simulink model "Cau3"  (R2021b)
settings: Solver=VariableStepAuto  StartTime=0.0  StopTime=inf  RelTol=1e-3
libraries: commsink2 x2, commutil2 x2, commdigbbndpm3 x2, commchan3 x1, commrandsrc3 x1
settings Model: Creator=ICTLAB  LastModifiedBy=ICTLAB
settings DataIOCC: ReturnWorkspaceOutputs=off

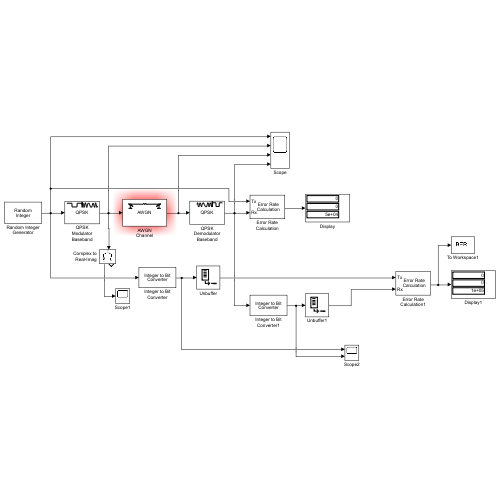
[thumbnail: Simulink's stored preview of the top-level diagram]
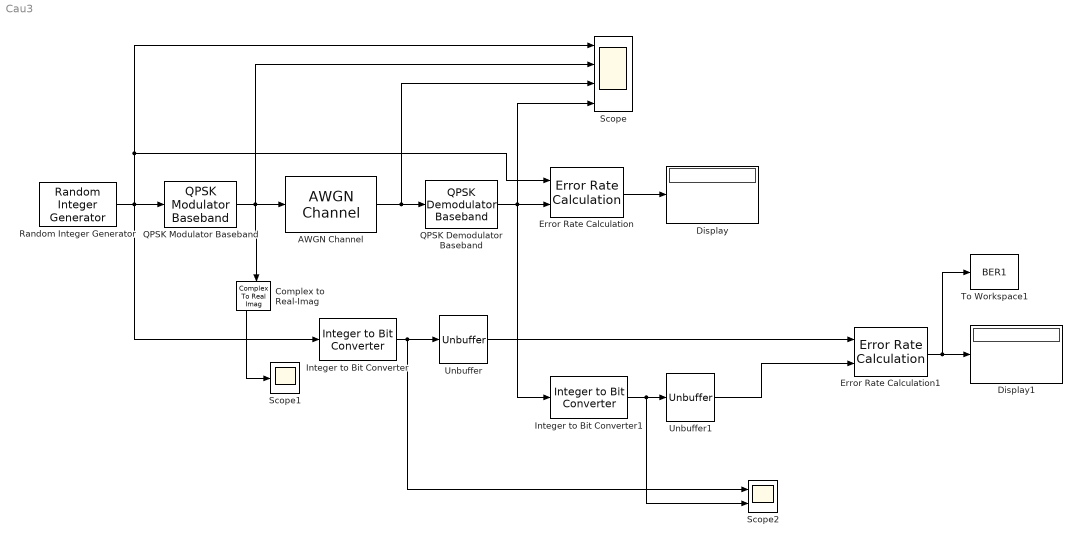
== system Cau3 ==
  AWGN Channel : commchan3/AWGN Channel  InputProcessing=Columns as channels (frame based)  seed=67  noiseMode="Signal to noise ratio  (Eb/No)"  EbNodB=EbNo  EsNodB=10  SNRdB=10  bitsPerSym=2  Ps=1  Tsym=1/1000  variance=1
  Complex to Real-Imag : ComplexToRealImag
  Display : Display
  Display1 : Display
  Error Rate Calculation : commsink2/Error Rate Calculation  N=0  st_delay=0  cp_mode=Entire frame  subframe=[]  PMode=Port  WsName=ErrorVec  RsMode2=off  stop=on  numErr=1e4  maxBits=1e5
  Error Rate Calculation1 : commsink2/Error Rate Calculation  N=0  st_delay=0  cp_mode=Entire frame  subframe=[]  PMode=Port  WsName=ErrorVec  RsMode2=off  stop=on  numErr=1e4  maxBits=1e5
  Integer to Bit Converter : commutil2/Integer to Bit Converter  nbits=2  signedInputValues=Unsigned  bitOrder=MSB first  outDtype=Inherit via internal rule
  Integer to Bit Converter1 : commutil2/Integer to Bit Converter  nbits=2  signedInputValues=Unsigned  bitOrder=MSB first  outDtype=Inherit via internal rule
  QPSK Demodulator Baseband : commdigbbndpm3/QPSK Demodulator Baseband  OutType=Integer  DecType=Hard decision  VarSource=Dialog  Variance=1  Dec=Gray  Ph=pi/4  outDtype1=Inherit via internal rule  outDtype2=Inherit via internal rule  derotateFactorWordLen=16  derotateFactorDataTypeStr=Inherit: Same word length as input  derotateFactorLastDataTypeStr=Inherit: Same word length as input
  QPSK Modulator Baseband : commdigbbndpm3/QPSK Modulator Baseband  InType=Integer  Enc=Gray  Ph=pi/4  outDtype=double  outWordLen=16  outUDDataType=sfix(16)  outFracLenMode=Best precision  outFracLen=15  outDataTypeStr=double  outLastDataTypeStr=double
  Random Integer Generator : commrandsrc3/Random Integer Generator  SetSize=4  SeedSource=Auto  Seed=0  SampleTime=1/1000  SamplesPerFrame=1  OutputDataType=double  SimulateUsing=Interpreted execution
  Scope : Scope  NumInputPorts=4
  Scope1 : Scope
  Scope2 : Scope  NumInputPorts=2
  To Workspace1 : ToWorkspace  VariableName=BER1  SampleTime=-1
      settings: MaxDataPoints=1
  Unbuffer : Unbuffer
  Unbuffer1 : Unbuffer
  wires:
  Random Integer Generator/1 -> QPSK Modulator Baseband/1, Integer to Bit Converter/1, Scope/1, Error Rate Calculation/1
  QPSK Modulator Baseband/1 -> Complex to Real-Imag/1, AWGN Channel/1, Scope/2
  AWGN Channel/1 -> QPSK Demodulator Baseband/1, Scope/3
  QPSK Demodulator Baseband/1 -> Scope/4, Integer to Bit Converter1/1, Error Rate Calculation/2
  Error Rate Calculation/1 -> Display/1
  Integer to Bit Converter/1 -> Scope2/1, Unbuffer/1
  Unbuffer/1 -> Error Rate Calculation1/1
  Integer to Bit Converter1/1 -> Scope2/2, Unbuffer1/1
  Unbuffer1/1 -> Error Rate Calculation1/2
  Error Rate Calculation1/1 -> To Workspace1/1, Display1/1
  Complex to Real-Imag/1 -> Scope1/1
